simulink model "hdl_learn_mlfcn"  (R2025b)
settings: Solver=FixedStepDiscrete  StartTime=0.0  StopTime=0.02  FixedStep=0.0001  RelTol=1e-3
libraries: simulink x1
settings Model: DataTypeOverride=Off  Creator=kimsteph  LastModifiedBy=kimsteph
settings OptimizationCC: BlockReduction=off  ConditionallyExecuteInputs=off  DefaultParameterBehavior=Inlined  InheritOutputTypeSmallerThanSingle=on
settings DebuggingCC: ArtificialAlgebraicLoopMsg=error  SingleTaskRateTransMsg=error
settings HardwareCC: ProdBitPerPointer=32.0  ProdBitPerSizeT=32.0  ProdBitPerPtrDiffT=32.0  ProdLargestAtomicFloat=None  ProdIntDivRoundTo=Undefined  ProdEndianess=Unspecified  ProdWordSize=32.0  ProdHWDeviceType=ASIC/FPGA->ASIC/FPGA  TargetBitPerPointer=64.0  TargetBitPerSizeT=64.0  TargetBitPerPtrDiffT=64.0  TargetLongLongMode=on  TargetIntDivRoundTo=Zero  TargetEndianess=LittleEndian  TargetWordSize=64.0  TargetHWDeviceType=Custom Processor->MATLAB Host Computer  ProdEqTarget=off

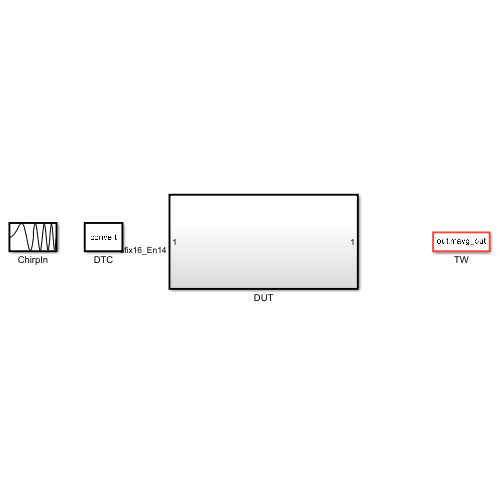
[thumbnail: Simulink's stored preview of the top-level diagram]
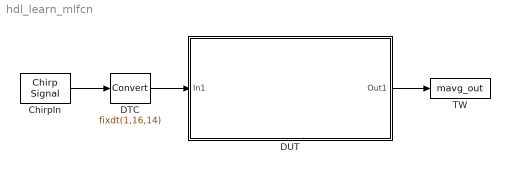
== system hdl_learn_mlfcn ==
  ChirpIn : simulink/Sources/Chirp Signal  f1=100  T=0.02  f2=3000
  DTC : DataTypeConversion  OutDataTypeStr=fixdt(1,16,14)  RndMeth=Nearest  SaturateOnIntegerOverflow=off
  DUT : Subsystem
  TW : ToWorkspace  VariableName=mavg_out  SaveFormat=Timeseries  SampleTime=-1
  wires:
  DTC/1 -> DUT/1(In1)
  ChirpIn/1 -> DTC/1
  DUT/1(Out1) -> TW/1

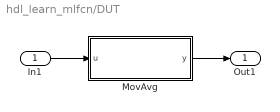
== system hdl_learn_mlfcn/DUT ==
  In1 : Inport  OutDataTypeStr=fixdt(1,16,14)
  MovAvg : MATLAB Function  TreatAsAtomicUnit=on
  Out1 : Outport
  wires:
  In1/1 -> MovAvg/1(u)
  MovAvg/1(y) -> Out1/1

== matlab function hdl_learn_mlfcn/DUT/MovAvg ==
  data: u input; y output
function y = fcn(u)
% 4-tap Moving Average Filter (HDL compatible)
% Persistent variables for delay line
persistent d1 d2 d3
if isempty(d1)
    d1 = fi(0, 1, 16, 14);
    d2 = fi(0, 1, 16, 14);
    d3 = fi(0, 1, 16, 14);
end

% Compute average: (u + d1 + d2 + d3) / 4
sum_val = fi(u, 1, 18, 14) + fi(d1, 1, 18, 14) + fi(d2, 1, 18, 14) + fi(d3, 1, 18, 14);
y = fi(bitsra(sum_val, 2), 1, 16, 14);  % divide by 4 via shift

% Shift delay line
d3 = d2;
d2 = d1;
d1 = u;
